simulink model "Lab6_Optimised_simulink"  (R2024b)
settings: Solver=FixedStepDiscrete  StartTime=0.0  StopTime=stop  RelTol=1e-3
values from neighbouring files (symbols this model uses):
  Ts = 1e-6    (= 1e-06)    [Lab6_matlab.m]
libraries: hdlsllib x8
settings Model: Creator=uqpnanth  LastModifiedBy=adubu
settings SolverCC: AlgebraicLoopSolver=TrustRegion
settings OptimizationCC: BlockReduction=off  ConditionallyExecuteInputs=off  DefaultParameterBehavior=Inlined
settings DebuggingCC: AlgebraicLoopMsg=error  InheritedTsInSrcMsg=error  SingleTaskRateTransMsg=error  UnconnectedInputMsg=warning  UnconnectedOutputMsg=warning  UnconnectedLineMsg=warning
settings HardwareCC: ProdBitPerPointer=32  ProdBitPerSizeT=32  ProdBitPerPtrDiffT=32  ProdLargestAtomicFloat=None  ProdIntDivRoundTo=Undefined  ProdEndianess=Unspecified  ProdWordSize=32  ProdHWDeviceType=ASIC/FPGA->ASIC/FPGA  TargetBitPerPointer=64  TargetBitPerSizeT=64  TargetBitPerPtrDiffT=64  TargetLongLongMode=on  TargetIntDivRoundTo=Zero  TargetEndianess=LittleEndian  TargetWordSize=64  TargetHWDeviceType=Custom Processor->MATLAB Host Computer  ProdEqTarget=off
settings ModelReferenceCC: EnableRefExpFcnMdlSchedulingChecks=on
settings RTWCC: GPUComputeCapability=3.5

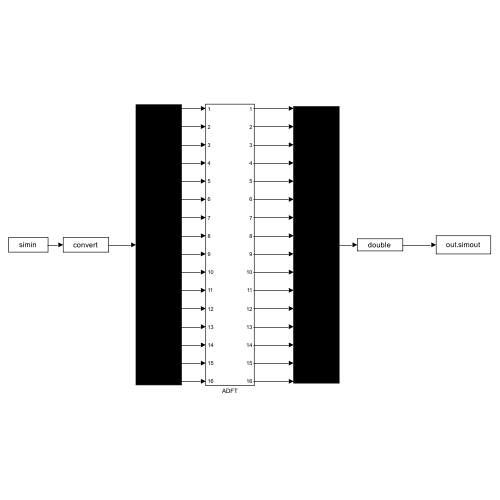
[thumbnail: Simulink's stored preview of the top-level diagram]
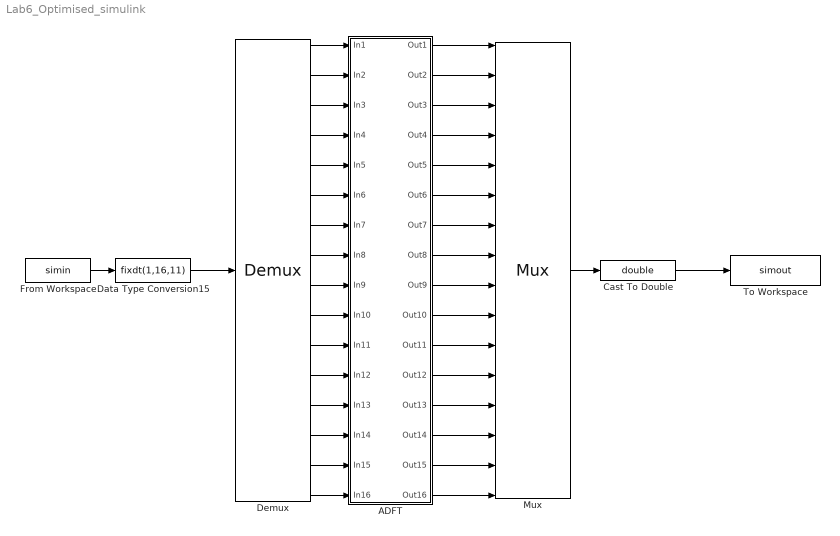
== system Lab6_Optimised_simulink ==
  ADFT : Subsystem
  Cast To Double : DataTypeConversion  OutDataTypeStr=double  SaturateOnIntegerOverflow=off  RndMeth=Floor
  Data Type Conversion15 : DataTypeConversion  OutDataTypeStr=fixdt(1,16,11)  RndMeth=Nearest
  Demux : Demux  Outputs=16
  From Workspace : FromWorkspace  VariableName=simin  SampleTime=Ts  OutputAfterFinalValue=Holding final value
  Mux : Mux  Inputs=16
  To Workspace : ToWorkspace  VariableName=simout  SampleTime=-1
  wires:
  Mux/1 -> Cast To Double/1
  ADFT/1(Out1) -> Mux/1
  ADFT/2(Out2) -> Mux/2
  ADFT/3(Out3) -> Mux/3
  ADFT/4(Out4) -> Mux/4
  ADFT/7(Out7) -> Mux/7
  ADFT/8(Out8) -> Mux/8
  ADFT/6(Out6) -> Mux/6
  ADFT/5(Out5) -> Mux/5
  ADFT/12(Out12) -> Mux/12
  ADFT/9(Out9) -> Mux/9
  ADFT/10(Out10) -> Mux/10
  ADFT/11(Out11) -> Mux/11
  ADFT/15(Out15) -> Mux/15
  ADFT/14(Out14) -> Mux/14
  ADFT/13(Out13) -> Mux/13
  ADFT/16(Out16) -> Mux/16
  Demux/1 -> ADFT/1(In1)
  Demux/2 -> ADFT/2(In2)
  Demux/3 -> ADFT/3(In3)
  Demux/4 -> ADFT/4(In4)
  Demux/6 -> ADFT/6(In6)
  Demux/7 -> ADFT/7(In7)
  Demux/8 -> ADFT/8(In8)
  Demux/5 -> ADFT/5(In5)
  Demux/9 -> ADFT/9(In9)
  Demux/11 -> ADFT/11(In11)
  Demux/10 -> ADFT/10(In10)
  Demux/12 -> ADFT/12(In12)
  Demux/15 -> ADFT/15(In15)
  Demux/14 -> ADFT/14(In14)
  Demux/13 -> ADFT/13(In13)
  From Workspace/1 -> Data Type Conversion15/1
  Data Type Conversion15/1 -> Demux/1
  Cast To Double/1 -> To Workspace/1
  Demux/16 -> ADFT/16(In16)

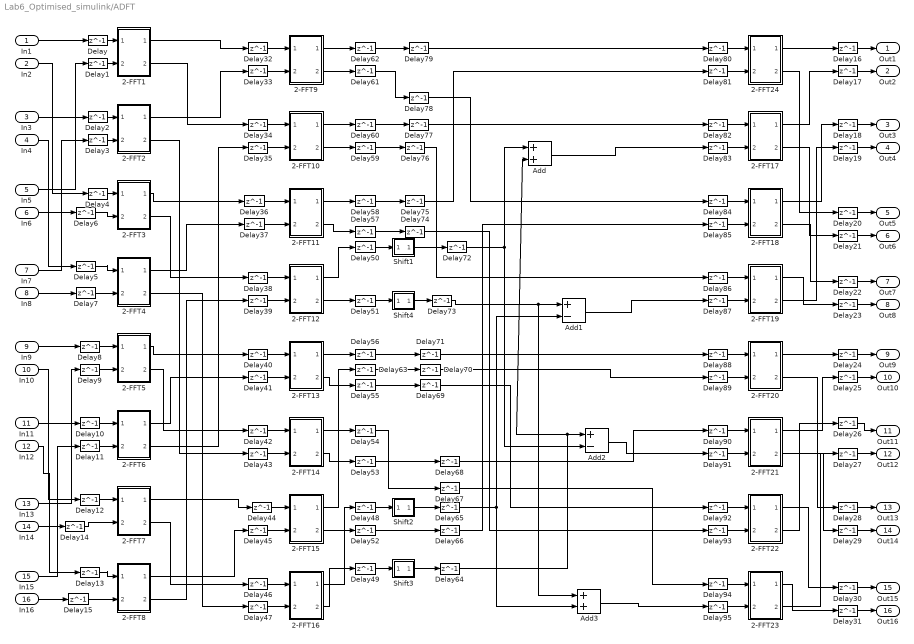
== system Lab6_Optimised_simulink/ADFT ==
  In1 : Inport
  In2 : Inport  Port=2
  In3 : Inport  Port=3
  In4 : Inport  Port=4
  In5 : Inport  Port=5
  In6 : Inport  Port=6
  In7 : Inport  Port=7
  In8 : Inport  Port=8
  In9 : Inport  Port=9
  In10 : Inport  Port=10
  In11 : Inport  Port=11
  In12 : Inport  Port=12
  In13 : Inport  Port=13
  In14 : Inport  Port=14
  In15 : Inport  Port=15
  In16 : Inport  Port=16
  2-FFT1 : Subsystem
  2-FFT10 : Subsystem
  2-FFT11 : Subsystem
  2-FFT12 : Subsystem
  2-FFT13 : Subsystem
  2-FFT14 : Subsystem
  2-FFT15 : Subsystem
  2-FFT16 : Subsystem
  2-FFT17 : Subsystem
  2-FFT18 : Subsystem
  2-FFT19 : Subsystem
  2-FFT2 : Subsystem
  2-FFT20 : Subsystem
  2-FFT21 : Subsystem
  2-FFT22 : Subsystem
  2-FFT23 : Subsystem
  2-FFT24 : Subsystem
  2-FFT3 : Subsystem
  2-FFT4 : Subsystem
  2-FFT5 : Subsystem
  2-FFT6 : Subsystem
  2-FFT7 : Subsystem
  2-FFT8 : Subsystem
  2-FFT9 : Subsystem
  Add : Sum  OutDataTypeStr=fixdt(1,W,D)
  Add1 : Sum  Inputs=+-  OutDataTypeStr=fixdt(1,W,D)
  Add2 : Sum  Inputs=+-  OutDataTypeStr=fixdt(1,W,D)
  Add3 : Sum  OutDataTypeStr=fixdt(1,W,D)
  Delay{,1..95} (96 alike) : Delay  DelayLength=1
  Shift1 : Subsystem
  Shift2 : Subsystem
  Shift3 : Subsystem
  Shift4 : Subsystem
  Out1 : Outport
  Out2 : Outport  Port=2
  Out3 : Outport  Port=3
  Out4 : Outport  Port=4
  Out5 : Outport  Port=5
  Out6 : Outport  Port=6
  Out7 : Outport  Port=7
  Out8 : Outport  Port=8
  Out9 : Outport  Port=9
  Out10 : Outport  Port=10
  Out11 : Outport  Port=11
  Out12 : Outport  Port=12
  Out13 : Outport  Port=13
  Out14 : Outport  Port=14
  Out15 : Outport  Port=15
  Out16 : Outport  Port=16
  wires:
  In1/1 -> Delay/1
  In5/1 -> Delay1/1
  In3/1 -> Delay2/1
  In7/1 -> Delay3/1
  In2/1 -> Delay4/1
  In6/1 -> Delay6/1
  In4/1 -> Delay5/1
  In8/1 -> Delay7/1
  In9/1 -> Delay8/1
  In13/1 -> Delay9/1
  In11/1 -> Delay10/1
  In15/1 -> Delay11/1
  In10/1 -> Delay12/1
  In14/1 -> Delay14/1
  In12/1 -> Delay13/1
  In16/1 -> Delay15/1
  2-FFT1/1(Out1) -> Delay32/1
  2-FFT2/1(Out1) -> Delay33/1
  2-FFT1/2(Out2) -> Delay34/1
  2-FFT6/2(Out2) -> Delay35/1
  2-FFT3/1(Out1) -> Delay36/1
  2-FFT4/1(Out1) -> Delay37/1
  2-FFT3/2(Out2) -> Delay38/1
  2-FFT8/2(Out2) -> Delay39/1
  2-FFT5/1(Out1) -> Delay40/1
  2-FFT6/1(Out1) -> Delay41/1
  2-FFT5/2(Out2) -> Delay42/1
  2-FFT2/2(Out2) -> Delay43/1
  2-FFT7/1(Out1) -> Delay44/1
  2-FFT8/1(Out1) -> Delay45/1
  2-FFT7/2(Out2) -> Delay46/1
  2-FFT4/2(Out2) -> Delay47/1
  2-FFT9/1(Out1) -> Delay62/1
  2-FFT11/1(Out1) -> Delay58/1
  2-FFT10/1(Out1) -> Delay60/1
  Add/1 -> Delay83/1
  2-FFT9/2(Out2) -> Delay61/1
  2-FFT15/2(Out2) -> Delay52/1
  2-FFT10/2(Out2) -> Delay59/1
  2-FFT12/1(Out1) -> Delay50/1
  2-FFT12/2(Out2) -> Delay51/1
  2-FFT16/1(Out1) -> Delay48/1
  2-FFT16/2(Out2) -> Delay49/1
  Shift1/1(Out1) -> Delay72/1
  Shift4/1(Out1) -> Delay73/1
  Shift2/1(Out1) -> Delay65/1
  Shift3/1(Out1) -> Delay64/1
  Add1/1 -> Delay87/1
  2-FFT13/1(Out1) -> Delay56/1
  2-FFT15/1(Out1) -> Delay63/1
  2-FFT14/2(Out2) -> Delay53/1
  Add2/1 -> Delay91/1
  2-FFT13/2(Out2) -> Delay55/1
  2-FFT11/2(Out2) -> Delay57/1
  2-FFT14/1(Out1) -> Delay54/1
  Add3/1 -> Delay95/1
  2-FFT24/1(Out1) -> Delay16/1
  2-FFT17/1(Out1) -> Delay17/1
  2-FFT18/1(Out1) -> Delay18/1
  2-FFT19/2(Out2) -> Delay19/1
  2-FFT24/2(Out2) -> Delay20/1
  2-FFT17/2(Out2) -> Delay21/1
  2-FFT18/2(Out2) -> Delay22/1
  2-FFT19/1(Out1) -> Delay23/1
  2-FFT20/1(Out1) -> Delay24/1
  2-FFT21/1(Out1) -> Delay25/1
  2-FFT22/2(Out2) -> Delay26/1
  2-FFT23/2(Out2) -> Delay27/1
  2-FFT20/2(Out2) -> Delay28/1
  2-FFT21/2(Out2) -> Delay29/1
  2-FFT22/1(Out1) -> Delay30/1
  2-FFT23/1(Out1) -> Delay31/1
  Delay/1 -> 2-FFT1/1(In1)
  Delay3/1 -> 2-FFT2/2(In2)
  Delay2/1 -> 2-FFT2/1(In1)
  Delay1/1 -> 2-FFT1/2(In2)
  Delay4/1 -> 2-FFT3/1(In1)
  Delay5/1 -> 2-FFT4/1(In1)
  Delay6/1 -> 2-FFT3/2(In2)
  Delay7/1 -> 2-FFT4/2(In2)
  Delay8/1 -> 2-FFT5/1(In1)
  Delay10/1 -> 2-FFT6/1(In1)
  Delay11/1 -> 2-FFT6/2(In2)
  Delay12/1 -> 2-FFT7/1(In1)
  Delay15/1 -> 2-FFT8/2(In2)
  Delay9/1 -> 2-FFT5/2(In2)
  Delay14/1 -> 2-FFT7/2(In2)
  Delay13/1 -> 2-FFT8/1(In1)
  Delay16/1 -> Out1/1
  Delay17/1 -> Out2/1
  Delay18/1 -> Out3/1
  Delay19/1 -> Out4/1
  Delay20/1 -> Out5/1
  Delay21/1 -> Out6/1
  Delay22/1 -> Out7/1
  Delay24/1 -> Out9/1
  Delay25/1 -> Out10/1
  Delay23/1 -> Out8/1
  Delay27/1 -> Out12/1
  Delay26/1 -> Out11/1
  Delay29/1 -> Out14/1
  Delay28/1 -> Out13/1
  Delay31/1 -> Out16/1
  Delay30/1 -> Out15/1
  Delay34/1 -> 2-FFT10/1(In1)
  Delay32/1 -> 2-FFT9/1(In1)
  Delay46/1 -> 2-FFT16/1(In1)
  Delay35/1 -> 2-FFT10/2(In2)
  Delay39/1 -> 2-FFT12/2(In2)
  Delay38/1 -> 2-FFT12/1(In1)
  Delay43/1 -> 2-FFT14/2(In2)
  Delay47/1 -> 2-FFT16/2(In2)
  Delay45/1 -> 2-FFT15/2(In2)
  Delay33/1 -> 2-FFT9/2(In2)
  Delay41/1 -> 2-FFT13/2(In2)
  Delay36/1 -> 2-FFT11/1(In1)
  Delay37/1 -> 2-FFT11/2(In2)
  Delay40/1 -> 2-FFT13/1(In1)
  Delay42/1 -> 2-FFT14/1(In1)
  Delay44/1 -> 2-FFT15/1(In1)
  Delay48/1 -> Shift2/1(In1)
  Delay49/1 -> Shift3/1(In1)
  Delay50/1 -> Shift1/1(In1)
  Delay51/1 -> Shift4/1(In1)
  Delay52/1 -> Delay66/1
  Delay53/1 -> Delay68/1
  Delay54/1 -> Delay67/1
  Delay55/1 -> Delay69/1
  Delay56/1 -> Delay71/1
  Delay57/1 -> Delay74/1
  Delay58/1 -> Delay75/1
  Delay59/1 -> Delay76/1
  Delay60/1 -> Delay77/1
  Delay61/1 -> Delay78/1
  Delay62/1 -> Delay79/1
  Delay63/1 -> Delay70/1
  Delay64/1 -> Add2/1, Add/2
  Delay65/1 -> Add3/2, Add1/2
  Delay66/1 -> Delay85/1
  Delay67/1 -> Delay94/1
  Delay68/1 -> Delay90/1
  Delay69/1 -> Delay92/1
  Delay70/1 -> Delay89/1
  Delay71/1 -> Delay88/1
  Delay72/1 -> Add2/2, Add/1
  Delay73/1 -> Add1/1, Add3/1
  Delay74/1 -> Delay93/1
  Delay75/1 -> Delay81/1
  Delay76/1 -> Delay86/1
  Delay77/1 -> Delay82/1
  Delay78/1 -> Delay84/1
  Delay79/1 -> Delay80/1
  Delay83/1 -> 2-FFT17/2(In2)
  Delay91/1 -> 2-FFT21/2(In2)
  Delay93/1 -> 2-FFT22/2(In2)
  Delay89/1 -> 2-FFT20/2(In2)
  Delay87/1 -> 2-FFT19/2(In2)
  Delay80/1 -> 2-FFT24/1(In1)
  Delay81/1 -> 2-FFT24/2(In2)
  Delay86/1 -> 2-FFT19/1(In1)
  Delay82/1 -> 2-FFT17/1(In1)
  Delay88/1 -> 2-FFT20/1(In1)
  Delay94/1 -> 2-FFT23/1(In1)
  Delay95/1 -> 2-FFT23/2(In2)
  Delay92/1 -> 2-FFT22/1(In1)
  Delay84/1 -> 2-FFT18/1(In1)
  Delay85/1 -> 2-FFT18/2(In2)
  Delay90/1 -> 2-FFT21/1(In1)

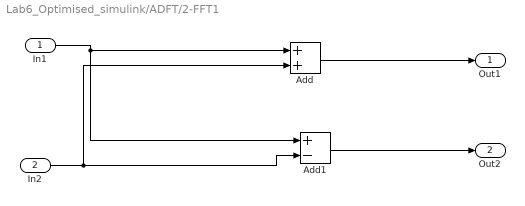
== system Lab6_Optimised_simulink/ADFT/2-FFT1 ==
  In1 : Inport
  In2 : Inport  Port=2
  Add : Sum  OutDataTypeStr=fixdt(1,W,D)
  Add1 : Sum  Inputs=+-  OutDataTypeStr=fixdt(1,W,D)
  Out1 : Outport
  Out2 : Outport  Port=2
  wires:
  In1/1 -> Add1/1, Add/1
  In2/1 -> Add1/2, Add/2
  Add/1 -> Out1/1
  Add1/1 -> Out2/1

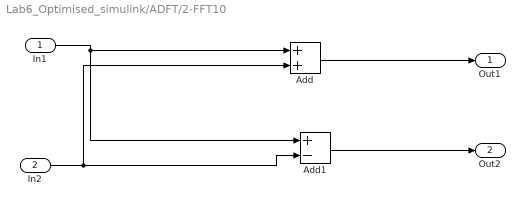
== system Lab6_Optimised_simulink/ADFT/2-FFT10 ==
  In1 : Inport
  In2 : Inport  Port=2
  Add : Sum  OutDataTypeStr=fixdt(1,W,D)
  Add1 : Sum  Inputs=+-  OutDataTypeStr=fixdt(1,W,D)
  Out1 : Outport
  Out2 : Outport  Port=2
  wires:
  In1/1 -> Add1/1, Add/1
  In2/1 -> Add1/2, Add/2
  Add/1 -> Out1/1
  Add1/1 -> Out2/1

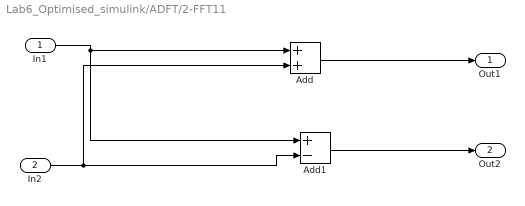
== system Lab6_Optimised_simulink/ADFT/2-FFT11 ==
  In1 : Inport
  In2 : Inport  Port=2
  Add : Sum  OutDataTypeStr=fixdt(1,W,D)
  Add1 : Sum  Inputs=+-  OutDataTypeStr=fixdt(1,W,D)
  Out1 : Outport
  Out2 : Outport  Port=2
  wires:
  In1/1 -> Add1/1, Add/1
  In2/1 -> Add1/2, Add/2
  Add/1 -> Out1/1
  Add1/1 -> Out2/1

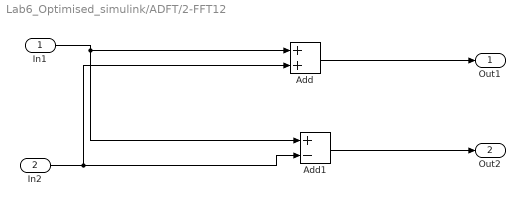
== system Lab6_Optimised_simulink/ADFT/2-FFT12 ==
  In1 : Inport
  In2 : Inport  Port=2
  Add : Sum  OutDataTypeStr=fixdt(1,W,D)
  Add1 : Sum  Inputs=+-  OutDataTypeStr=fixdt(1,W,D)
  Out1 : Outport
  Out2 : Outport  Port=2
  wires:
  In1/1 -> Add1/1, Add/1
  In2/1 -> Add1/2, Add/2
  Add/1 -> Out1/1
  Add1/1 -> Out2/1

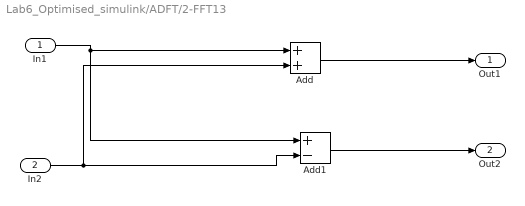
== system Lab6_Optimised_simulink/ADFT/2-FFT13 ==
  In1 : Inport
  In2 : Inport  Port=2
  Add : Sum  OutDataTypeStr=fixdt(1,W,D)
  Add1 : Sum  Inputs=+-  OutDataTypeStr=fixdt(1,W,D)
  Out1 : Outport
  Out2 : Outport  Port=2
  wires:
  In1/1 -> Add1/1, Add/1
  In2/1 -> Add1/2, Add/2
  Add/1 -> Out1/1
  Add1/1 -> Out2/1

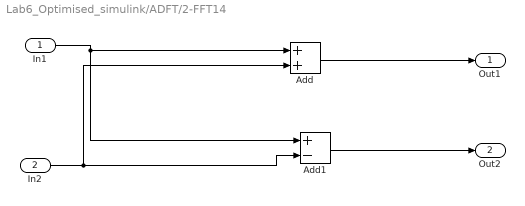
== system Lab6_Optimised_simulink/ADFT/2-FFT14 ==
  In1 : Inport
  In2 : Inport  Port=2
  Add : Sum  OutDataTypeStr=fixdt(1,W,D)
  Add1 : Sum  Inputs=+-  OutDataTypeStr=fixdt(1,W,D)
  Out1 : Outport
  Out2 : Outport  Port=2
  wires:
  In1/1 -> Add1/1, Add/1
  In2/1 -> Add1/2, Add/2
  Add/1 -> Out1/1
  Add1/1 -> Out2/1

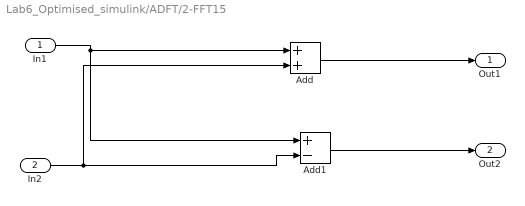
== system Lab6_Optimised_simulink/ADFT/2-FFT15 ==
  In1 : Inport
  In2 : Inport  Port=2
  Add : Sum  OutDataTypeStr=fixdt(1,W,D)
  Add1 : Sum  Inputs=+-  OutDataTypeStr=fixdt(1,W,D)
  Out1 : Outport
  Out2 : Outport  Port=2
  wires:
  In1/1 -> Add1/1, Add/1
  In2/1 -> Add1/2, Add/2
  Add/1 -> Out1/1
  Add1/1 -> Out2/1

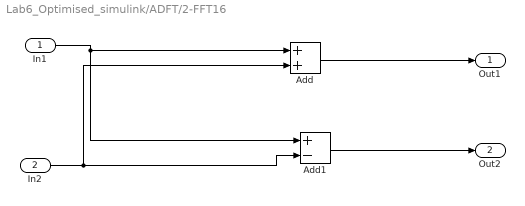
== system Lab6_Optimised_simulink/ADFT/2-FFT16 ==
  In1 : Inport
  In2 : Inport  Port=2
  Add : Sum  OutDataTypeStr=fixdt(1,W,D)
  Add1 : Sum  Inputs=+-  OutDataTypeStr=fixdt(1,W,D)
  Out1 : Outport
  Out2 : Outport  Port=2
  wires:
  In1/1 -> Add1/1, Add/1
  In2/1 -> Add1/2, Add/2
  Add/1 -> Out1/1
  Add1/1 -> Out2/1

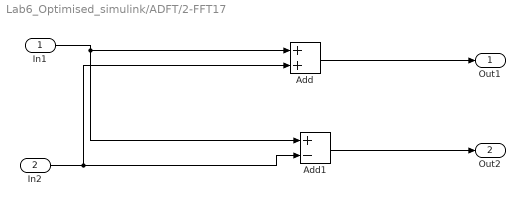
== system Lab6_Optimised_simulink/ADFT/2-FFT17 ==
  In1 : Inport
  In2 : Inport  Port=2
  Add : Sum  OutDataTypeStr=fixdt(1,W,D)
  Add1 : Sum  Inputs=+-  OutDataTypeStr=fixdt(1,W,D)
  Out1 : Outport
  Out2 : Outport  Port=2
  wires:
  In1/1 -> Add1/1, Add/1
  In2/1 -> Add1/2, Add/2
  Add/1 -> Out1/1
  Add1/1 -> Out2/1

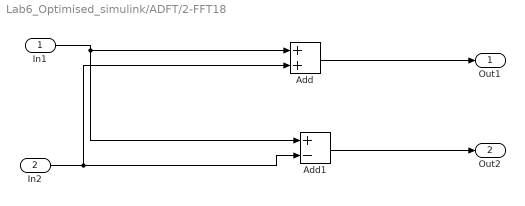
== system Lab6_Optimised_simulink/ADFT/2-FFT18 ==
  In1 : Inport
  In2 : Inport  Port=2
  Add : Sum  OutDataTypeStr=fixdt(1,W,D)
  Add1 : Sum  Inputs=+-  OutDataTypeStr=fixdt(1,W,D)
  Out1 : Outport
  Out2 : Outport  Port=2
  wires:
  In1/1 -> Add1/1, Add/1
  In2/1 -> Add1/2, Add/2
  Add/1 -> Out1/1
  Add1/1 -> Out2/1

== system Lab6_Optimised_simulink/ADFT/2-FFT19 ==
  In1 : Inport
  In2 : Inport  Port=2
  Add : Sum  OutDataTypeStr=fixdt(1,W,D)
  Add1 : Sum  Inputs=+-  OutDataTypeStr=fixdt(1,W,D)
  Out1 : Outport
  Out2 : Outport  Port=2
  wires:
  In1/1 -> Add1/1, Add/1
  In2/1 -> Add1/2, Add/2
  Add/1 -> Out1/1
  Add1/1 -> Out2/1

== system Lab6_Optimised_simulink/ADFT/2-FFT2 ==
  In1 : Inport
  In2 : Inport  Port=2
  Add : Sum  OutDataTypeStr=fixdt(1,W,D)
  Add1 : Sum  Inputs=+-  OutDataTypeStr=fixdt(1,W,D)
  Out1 : Outport
  Out2 : Outport  Port=2
  wires:
  In1/1 -> Add1/1, Add/1
  In2/1 -> Add1/2, Add/2
  Add/1 -> Out1/1
  Add1/1 -> Out2/1

== system Lab6_Optimised_simulink/ADFT/2-FFT20 ==
  In1 : Inport
  In2 : Inport  Port=2
  Add : Sum  OutDataTypeStr=fixdt(1,W,D)
  Add1 : Sum  Inputs=+-  OutDataTypeStr=fixdt(1,W,D)
  Out1 : Outport
  Out2 : Outport  Port=2
  wires:
  In1/1 -> Add1/1, Add/1
  In2/1 -> Add1/2, Add/2
  Add/1 -> Out1/1
  Add1/1 -> Out2/1

== system Lab6_Optimised_simulink/ADFT/2-FFT21 ==
  In1 : Inport
  In2 : Inport  Port=2
  Add : Sum  OutDataTypeStr=fixdt(1,W,D)
  Add1 : Sum  Inputs=+-  OutDataTypeStr=fixdt(1,W,D)
  Out1 : Outport
  Out2 : Outport  Port=2
  wires:
  In1/1 -> Add1/1, Add/1
  In2/1 -> Add1/2, Add/2
  Add/1 -> Out1/1
  Add1/1 -> Out2/1

== system Lab6_Optimised_simulink/ADFT/2-FFT22 ==
  In1 : Inport
  In2 : Inport  Port=2
  Add : Sum  OutDataTypeStr=fixdt(1,W,D)
  Add1 : Sum  Inputs=+-  OutDataTypeStr=fixdt(1,W,D)
  Out1 : Outport
  Out2 : Outport  Port=2
  wires:
  In1/1 -> Add1/1, Add/1
  In2/1 -> Add1/2, Add/2
  Add/1 -> Out1/1
  Add1/1 -> Out2/1

== system Lab6_Optimised_simulink/ADFT/2-FFT23 ==
  In1 : Inport
  In2 : Inport  Port=2
  Add : Sum  OutDataTypeStr=fixdt(1,W,D)
  Add1 : Sum  Inputs=+-  OutDataTypeStr=fixdt(1,W,D)
  Out1 : Outport
  Out2 : Outport  Port=2
  wires:
  In1/1 -> Add1/1, Add/1
  In2/1 -> Add1/2, Add/2
  Add/1 -> Out1/1
  Add1/1 -> Out2/1

== system Lab6_Optimised_simulink/ADFT/2-FFT24 ==
  In1 : Inport
  In2 : Inport  Port=2
  Add : Sum  OutDataTypeStr=fixdt(1,W,D)
  Add1 : Sum  Inputs=+-  OutDataTypeStr=fixdt(1,W,D)
  Out1 : Outport
  Out2 : Outport  Port=2
  wires:
  In1/1 -> Add1/1, Add/1
  In2/1 -> Add1/2, Add/2
  Add/1 -> Out1/1
  Add1/1 -> Out2/1

== system Lab6_Optimised_simulink/ADFT/2-FFT3 ==
  In1 : Inport
  In2 : Inport  Port=2
  Add : Sum  OutDataTypeStr=fixdt(1,W,D)
  Add1 : Sum  Inputs=+-  OutDataTypeStr=fixdt(1,W,D)
  Out1 : Outport
  Out2 : Outport  Port=2
  wires:
  In1/1 -> Add1/1, Add/1
  In2/1 -> Add1/2, Add/2
  Add/1 -> Out1/1
  Add1/1 -> Out2/1

== system Lab6_Optimised_simulink/ADFT/2-FFT4 ==
  In1 : Inport
  In2 : Inport  Port=2
  Add : Sum  OutDataTypeStr=fixdt(1,W,D)
  Add1 : Sum  Inputs=+-  OutDataTypeStr=fixdt(1,W,D)
  Out1 : Outport
  Out2 : Outport  Port=2
  wires:
  In1/1 -> Add1/1, Add/1
  In2/1 -> Add1/2, Add/2
  Add/1 -> Out1/1
  Add1/1 -> Out2/1

== system Lab6_Optimised_simulink/ADFT/2-FFT5 ==
  In1 : Inport
  In2 : Inport  Port=2
  Add : Sum  OutDataTypeStr=fixdt(1,W,D)
  Add1 : Sum  Inputs=+-  OutDataTypeStr=fixdt(1,W,D)
  Out1 : Outport
  Out2 : Outport  Port=2
  wires:
  In1/1 -> Add1/1, Add/1
  In2/1 -> Add1/2, Add/2
  Add/1 -> Out1/1
  Add1/1 -> Out2/1

== system Lab6_Optimised_simulink/ADFT/2-FFT6 ==
  In1 : Inport
  In2 : Inport  Port=2
  Add : Sum  OutDataTypeStr=fixdt(1,W,D)
  Add1 : Sum  Inputs=+-  OutDataTypeStr=fixdt(1,W,D)
  Out1 : Outport
  Out2 : Outport  Port=2
  wires:
  In1/1 -> Add1/1, Add/1
  In2/1 -> Add1/2, Add/2
  Add/1 -> Out1/1
  Add1/1 -> Out2/1

== system Lab6_Optimised_simulink/ADFT/2-FFT7 ==
  In1 : Inport
  In2 : Inport  Port=2
  Add : Sum  OutDataTypeStr=fixdt(1,W,D)
  Add1 : Sum  Inputs=+-  OutDataTypeStr=fixdt(1,W,D)
  Out1 : Outport
  Out2 : Outport  Port=2
  wires:
  In1/1 -> Add1/1, Add/1
  In2/1 -> Add1/2, Add/2
  Add/1 -> Out1/1
  Add1/1 -> Out2/1

== system Lab6_Optimised_simulink/ADFT/2-FFT8 ==
  In1 : Inport
  In2 : Inport  Port=2
  Add : Sum  OutDataTypeStr=fixdt(1,W,D)
  Add1 : Sum  Inputs=+-  OutDataTypeStr=fixdt(1,W,D)
  Out1 : Outport
  Out2 : Outport  Port=2
  wires:
  In1/1 -> Add1/1, Add/1
  In2/1 -> Add1/2, Add/2
  Add/1 -> Out1/1
  Add1/1 -> Out2/1

== system Lab6_Optimised_simulink/ADFT/2-FFT9 ==
  In1 : Inport
  In2 : Inport  Port=2
  Add : Sum  OutDataTypeStr=fixdt(1,W,D)
  Add1 : Sum  Inputs=+-  OutDataTypeStr=fixdt(1,W,D)
  Out1 : Outport
  Out2 : Outport  Port=2
  wires:
  In1/1 -> Add1/1, Add/1
  In2/1 -> Add1/2, Add/2
  Add/1 -> Out1/1
  Add1/1 -> Out2/1

== system Lab6_Optimised_simulink/ADFT/Shift1 ==
  In1 : Inport
  Add : Sum  OutDataTypeStr=fixdt(1,W,D)
  Bit Shift : hdlsllib/Logic and Bit Operations/Bit Shift  mode=Shift Right Arithmetic  N=1
  Bit Shift1 : hdlsllib/Logic and Bit Operations/Bit Shift  mode=Shift Right Arithmetic  N=2
  Out1 : Outport
  wires:
  Add/1 -> Out1/1
  Bit Shift1/1 -> Add/2
  Bit Shift/1 -> Add/1
  In1/1 -> Bit Shift1/1, Bit Shift/1

== system Lab6_Optimised_simulink/ADFT/Shift2 ==
  In1 : Inport
  Add : Sum  OutDataTypeStr=fixdt(1,W,D)
  Bit Shift : hdlsllib/Logic and Bit Operations/Bit Shift  mode=Shift Right Arithmetic  N=1
  Bit Shift1 : hdlsllib/Logic and Bit Operations/Bit Shift  mode=Shift Right Arithmetic  N=2
  Out1 : Outport
  wires:
  Add/1 -> Out1/1
  Bit Shift1/1 -> Add/2
  Bit Shift/1 -> Add/1
  In1/1 -> Bit Shift1/1, Bit Shift/1

== system Lab6_Optimised_simulink/ADFT/Shift3 ==
  In1 : Inport
  Add : Sum  OutDataTypeStr=fixdt(1,W,D)
  Bit Shift : hdlsllib/Logic and Bit Operations/Bit Shift  mode=Shift Right Arithmetic  N=1
  Bit Shift1 : hdlsllib/Logic and Bit Operations/Bit Shift  mode=Shift Right Arithmetic  N=2
  Out1 : Outport
  wires:
  Add/1 -> Out1/1
  Bit Shift1/1 -> Add/2
  Bit Shift/1 -> Add/1
  In1/1 -> Bit Shift1/1, Bit Shift/1

== system Lab6_Optimised_simulink/ADFT/Shift4 ==
  In1 : Inport
  Add : Sum  OutDataTypeStr=fixdt(1,W,D)
  Bit Shift : hdlsllib/Logic and Bit Operations/Bit Shift  mode=Shift Right Arithmetic  N=1
  Bit Shift1 : hdlsllib/Logic and Bit Operations/Bit Shift  mode=Shift Right Arithmetic  N=2
  Out1 : Outport
  wires:
  Add/1 -> Out1/1
  Bit Shift1/1 -> Add/2
  Bit Shift/1 -> Add/1
  In1/1 -> Bit Shift1/1, Bit Shift/1
